simulink model "grampc_R2008a"  (Simulink 7.1)
settings: Solver=FixedStepDiscrete  StartTime=0.0  StopTime=Tsim  FixedStep=grampc.param.dt  RelTol=1e-3
values from neighbouring files (symbols this model uses):
  grampc = grampc_init_Cmex()    [initData.m]
settings Model: Creator=kaepernick  LastModifiedBy=kaepernick
settings OptimizationCC: InitFltsAndDblsToZero=off
settings DebuggingCC: FcnCallInpInsideContextMsg=Enable All  StrictBusMsg=ErrorLevel1
settings CodeAppCC: CustomSymbolStrType=$N$R$M_T
settings GRTTargetCC: CombineOutputUpdateFcns=on  CPPClassGenCompliant=off

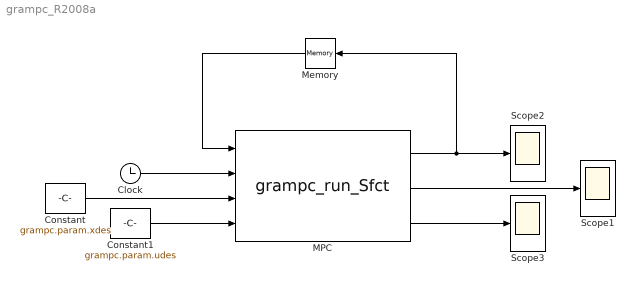
== system grampc_R2008a ==
  Clock : Clock
  Constant : Constant  Value=grampc.param.xdes
  Constant1 : Constant  Value=grampc.param.udes
  MPC : S-Function  FunctionName=grampc_run_Sfct  Parameters=grampc  EnableBusSupport=off
      mask Display:
      | port_label('input',1,'xk')
      | port_label('input',2,'tk')
      | port_label('input',3,'xdes')
      | port_label('input',4,'udes')
      | 
      | port_label('output',1,'xnext')
      | port_label('output',2,'unext')
      | port_label('output',3,'cost')
  Memory : Memory  Orientation=left  X0=grampc.param.xk
  Scope1 : Scope
  Scope2 : Scope
      settings: SaveName=ScopeData2
  Scope3 : Scope
  wires:
  MPC/1 -> Memory/1, Scope2/1
  MPC/2 -> Scope1/1
  MPC/3 -> Scope3/1
  Memory/1 -> MPC/1
  Clock/1 -> MPC/2
  Constant1/1 -> MPC/4
  Constant/1 -> MPC/3
